simulink model "keshe2fsk"  (R2023a)
settings: Solver=VariableStepAuto  StartTime=0.0  StopTime=10.0  RelTol=1e-3
libraries: dspfdesign x4, commchan3 x1, commrandsrc3 x1, simulink x1, commsink2 x1, dspsigops x1
settings Model: Creator=20896  LastModifiedBy=20896

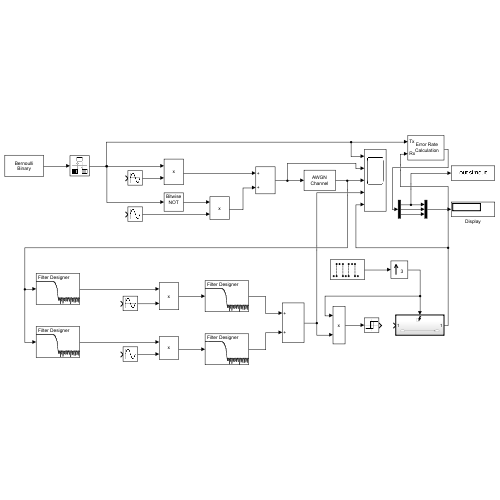
[thumbnail: Simulink's stored preview of the top-level diagram]
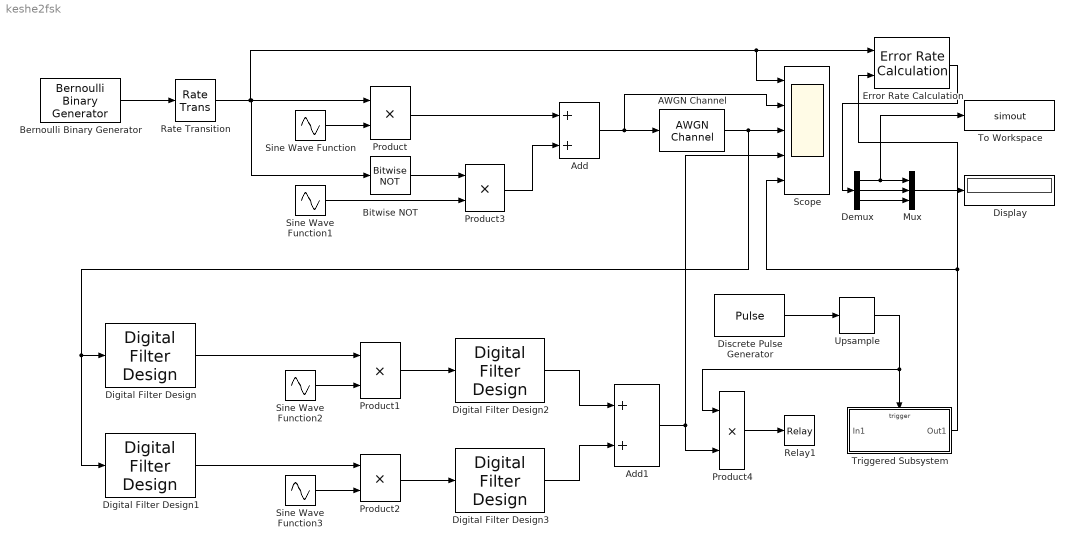
== system keshe2fsk ==
  AWGN Channel : commchan3/AWGN Channel  LegacyMode=off  NoiseMethod="Signal to noise ratio  (SNR)"  noiseMode="Signal to noise ratio  (SNR)"  EbNo=10  EsNo=10  SNR=10  BitsPerSymbol=1  SignalPower=1  SamplesPerSymbol=1  SymbolPeriod=1  VarianceSource=Parameter  Variance=1  RandomStream=Global stream  Seed=67  SimulateUsing=Code generation
  Add : Sum
  Add1 : Sum
  Bernoulli Binary Generator : commrandsrc3/Bernoulli Binary Generator  ProbabilityOfZero=0.5  SeedSource=Auto  Seed=0  SampleTime=1  SamplesPerFrame=1  OutputDataType=double  SimulateUsing=Interpreted execution
  Bitwise NOT : simulink/Logic and Bit Operations/Bitwise Operator  logicop=NOT  UseBitMask=off  BitMask=bin2dec('11011001')  BitMaskRealWorld=Stored Integer
      settings: LibrarySourceBlock=|
      | simulink/Quick Insert/Logic and Bit
      | Operations/Bitwise NOT
  Demux : Demux  Outputs=3
  Digital Filter Design{,1..3} (4 alike) : dspfdesign/Digital Filter Design  mwdsp_browser_bugfix_var=off
  Discrete Pulse Generator : DiscretePulseGenerator  Period=10  PulseWidth=5
  Display : Display
  Error Rate Calculation : commsink2/Error Rate Calculation  N=0  st_delay=0  cp_mode=Entire frame  subframe=[]  PMode=Port  WsName=ErrorVec  RsMode2=off  stop=off  numErr=100  maxBits=1e6
  Mux : Mux  Inputs=3
  Product{,1..4} (5 alike) : Product
  Rate Transition : RateTransition
  Relay1 : Relay
  Scope : Scope  NumInputPorts=5
  Sine Wave Function{,1..3} (4 alike) : Sin  TimeSource=Use external signal  SampleTime=0
  To Workspace : ToWorkspace  VariableName=simout  SaveFormat=Timeseries  SampleTime=-1
  Triggered Subsystem : Subsystem  TreatAsAtomicUnit=on
  Upsample : dspsigops/Upsample  FactorSource=Dialog parameter  N=3  Nmax=16  phase=0  InputProcessing=Columns as channels (frame based)  RateOptions=Enforce single-rate processing  ic=0  mode=Unused parameter value
  wires:
  Bernoulli Binary Generator/1 -> Rate Transition/1
  Rate Transition/1 -> Scope/1, Error Rate Calculation/1, Bitwise NOT/1, Product/1
  Sine Wave Function/1 -> Product/2
  Product/1 -> Add/1
  Bitwise NOT/1 -> Product3/1
  Sine Wave Function1/1 -> Product3/2
  Product3/1 -> Add/2
  Add/1 -> Scope/2, AWGN Channel/1
  Demux/1 -> To Workspace/1, Mux/1
  Demux/2 -> Mux/2
  Demux/3 -> Mux/3
  Mux/1 -> Display/1
  Digital Filter Design/1 -> Product1/1
  Sine Wave Function2/1 -> Product1/2
  Sine Wave Function3/1 -> Product2/2
  Digital Filter Design1/1 -> Product2/1
  Product1/1 -> Digital Filter Design2/1
  Product2/1 -> Digital Filter Design3/1
  Digital Filter Design2/1 -> Add1/1
  Digital Filter Design3/1 -> Add1/2
  Add1/1 -> Scope/4, Product4/2
  AWGN Channel/1 -> Digital Filter Design1/1, Digital Filter Design/1, Scope/3
  Product4/1 -> Relay1/1
  Discrete Pulse Generator/1 -> Upsample/1
  Upsample/1 -> Product4/1, Triggered Subsystem/Trigger
  Error Rate Calculation/1 -> Demux/1
  Triggered Subsystem/1(Out1) -> Scope/5, Error Rate Calculation/2

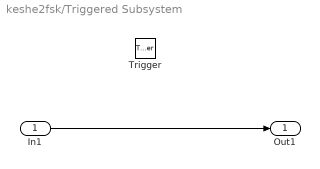
== system keshe2fsk/Triggered Subsystem ==
  In1 : Inport
  Trigger : TriggerPort  VariantControl=(inherit)
  Out1 : Outport
  wires:
  In1/1 -> Out1/1
